simulink model "timeVaryingPathModel3D"  (R2017b)
settings: Solver=VariableStepAuto  StartTime=0.0  StopTime=100  RelTol=1e-3  AbsTol=1e-7
settings Model: Creator=greenoctbass  LastModifiedBy=greenoctbass

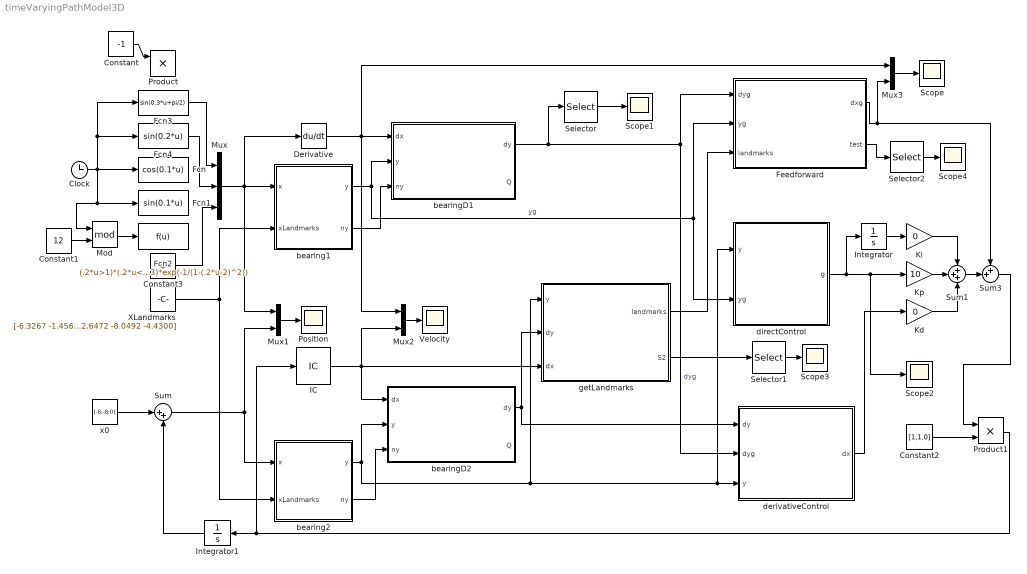
== system timeVaryingPathModel3D ==
  Clock : Clock
  Constant : Constant  Value=-1
  Constant1 : Constant  Value=12
  Constant2 : Constant  Value=[1,1,0]
  Constant3 : Constant  Value=0
  Derivative : Derivative
  Fcn : Fcn  Expr=cos(0.1*u)
  Fcn1 : Fcn  Expr=sin(0.1*u)
  Fcn2 : Fcn  Expr=(.2*u>1)*(.2*u<3)*exp(-1/(1-(.2*u-2)^2))
  Fcn3 : Fcn  Expr=sin(0.3*u+pi/2)
  Fcn4 : Fcn  Expr=sin(0.2*u)
  Feedforward : MATLAB Function  TreatAsAtomicUnit=on
  IC : InitialCondition  Value=[2,2,0]
  Integrator : Integrator
  Integrator1 : Integrator
  Kd : Gain  Gain=0
  Ki : Gain  Gain=0
  Kp : Gain  Gain=10
  Mod : Math  Operator=mod  SaturateOnIntegerOverflow=on
  Mux : Mux  Inputs=3
  Mux1 : Mux  Inputs=2
  Mux2 : Mux  Inputs=2
  Mux3 : Mux  Inputs=2
  Position : Scope
  Product : Product
  Product1 : Product
  Scope{,1..4} (5 alike) : Scope
  Selector : Selector  NumberOfDimensions=2  InputPortWidth=3  IndexOptions=Select all,Index vector (dialog)  Indices=[1 3],2  OutputSizes=1,1
  Selector1 : Selector  InputPortWidth=9  IndexOptions=Index vector (dialog)  Indices=[7 8 9]  OutputSizes=1
  Selector2 : Selector  InputPortWidth=3  IndexOptions=Select all  Indices=[1 2 3]  OutputSizes=1
  Sum : Sum  Inputs=|++
  Sum1 : Sum  Inputs=+++
  Sum3 : Sum  Inputs=++|
  Velocity : Scope
  XLandmarks : Constant  Value=[-6.3267 -1.4564 6.4309 -9.4093 -5.0582 -1.3374; -5.6740 9.4115 -2.6130 -6.1627 1.3438 2.2212; 8.1158 -7.4603 8.2675 2.6472 -8.0492 -4.4300]
  bearing1 : MATLAB Function  TreatAsAtomicUnit=on
  bearing2 : MATLAB Function  TreatAsAtomicUnit=on
  bearingD1 : MATLAB Function  TreatAsAtomicUnit=on
  bearingD2 : MATLAB Function  TreatAsAtomicUnit=on
  derivativeControl : MATLAB Function  TreatAsAtomicUnit=on
  directControl : MATLAB Function  TreatAsAtomicUnit=on
  getLandmarks : MATLAB Function  TreatAsAtomicUnit=on
  x0 : Constant  Value=[-8;-8;0]
  wires:
  XLandmarks/1 -> bearing2/2(xLandmarks), bearing1/2(xLandmarks)
  Mux/1 -> Mux1/1, Derivative/1, bearing1/1(x)
  bearing1/1(y) -> Feedforward/2(yg), directControl/2(yg), bearingD1/2(y)  "yg"
  Derivative/1 -> Mux3/1, bearingD1/1(dx), Mux2/1
  bearing1/2(ny) -> bearingD1/3(ny)
  x0/1 -> Sum/1
  Sum/1 -> Mux1/2, bearing2/1(x)
  bearing2/2(ny) -> bearingD2/3(ny)
  directControl/1(g) -> Integrator/1, Scope2/1, Kp/1
  Integrator/1 -> Ki/1
  Kp/1 -> Sum1/2
  Ki/1 -> Sum1/1
  Integrator1/1 -> Sum/2
  Mux1/1 -> Position/1
  derivativeControl/1(dx) -> Kd/1
  Mux2/1 -> Velocity/1
  bearing2/1(y) -> bearingD2/2(y), getLandmarks/1(y), directControl/1(y), derivativeControl/3(y)
  bearingD1/1(dy) -> derivativeControl/2(dyg), Feedforward/1(dyg), Selector/1  "dyg"
  bearingD2/1(dy) -> getLandmarks/2(dy), derivativeControl/1(dy)
  Kd/1 -> Sum1/3
  Selector/1 -> Scope1/1
  Mux3/1 -> Scope/1
  Product1/1 -> IC/1, Integrator1/1
  Clock/1 -> Mod/1, Fcn1/1, Fcn/1, Fcn4/1, Fcn3/1
  Constant1/1 -> Mod/2
  Constant/1 -> Product/1
  IC/1 -> getLandmarks/3(dx), Mux2/2, bearingD2/1(dx)
  Sum1/1 -> Sum3/2
  Feedforward/1(dxg) -> Sum3/1, Mux3/2
  Mod/1 -> Fcn2/1
  Fcn3/1 -> Mux/1
  Fcn4/1 -> Mux/2
  getLandmarks/1(landmarks) -> Feedforward/3(landmarks)
  getLandmarks/2(S2) -> Selector1/1
  Selector1/1 -> Scope3/1
  Sum3/1 -> Product1/1
  Constant2/1 -> Product1/2
  Constant3/1 -> Mux/3
  Selector2/1 -> Scope4/1
  Feedforward/2(test) -> Selector2/1

== matlab function timeVaryingPathModel3D/bearingD1 ==
  data: dx input; dy output; y input; ny input; Q output
%Compute derivative of bearing vectors
%function [dy,Q]=bearingComputeDerivative(dx,y,ny)
%Inputs
%   dx   derivative of robot's location
%   y   current bearings
%   ny  ranges corresponding to the bearings
%Output
%   dy  derivative of Y along v
%   Q   array of matrices such that dY=Q*v
function [dy,Q]=bearingComputeDerivative(dx,y,ny)
flagComputeQ=false;
if nargout>1
    flagComputeQ=true;
end
[d,Ny]=size(y);
dy=zeros(d,Ny);
if flagComputeQ
    Q=zeros(d,d,Ny);
end
I=eye(d);
for iY=1:Ny
    Qi=-inv(ny(iY))*(I-y(:,iY)*y(:,iY)');
    dy(:,iY)=Qi*dx;
    if flagComputeQ
        Q(:,:,iY)=Qi;
    end
end

== matlab function timeVaryingPathModel3D/bearing1 ==
  data: x input; y output; xLandmarks input; ny output
%Compute bearing information from base point and landmarks
%function [y,ny]=bearingCompute(x,xLandmarks)
%Inputs
%   x           coordinates of base point
%   xLandmarks  coordinates of landmarks
%Outputs
%   y       bearings
%   ny      ranges corresponding to the bearings
%
function [y,ny]=bearingCompute(x,xLandmarks)
Nx=size(x,2);
NxLandmarks=size(xLandmarks,2);
if Nx==1 && NxLandmarks>1
    z=x*ones(1,NxLandmarks);
elseif NxLandmarks==1 && Nx>1
    xLandmarks=xLandmarks*ones(1,Nx);
end
[y,ny]=cnormalize(xLandmarks-z);

== matlab function timeVaryingPathModel3D/bearing2 ==
  data: x input; y output; xLandmarks input; ny output
%Compute bearing information from base point and landmarks
%function [y,ny]=bearingCompute(x,xLandmarks)
%Inputs
%   x           coordinates of base point
%   xLandmarks  coordinates of landmarks
%Outputs
%   y       bearings
%   ny      ranges corresponding to the bearings
%
function [y,ny]=bearingCompute(x,xLandmarks)
Nx=size(x,2);
NxLandmarks=size(xLandmarks,2);
if Nx==1 && NxLandmarks>1
    z=x*ones(1,NxLandmarks);
elseif NxLandmarks==1 && Nx>1
    xLandmarks=xLandmarks*ones(1,Nx);
end
[y,ny]=cnormalize(xLandmarks-z);

== matlab function timeVaryingPathModel3D/bearingD2 ==
  data: dx input; dy output; y input; ny input; Q output
%Compute derivative of bearing vectors
%function [dy,Q]=bearingComputeDerivative(dx,y,ny)
%Inputs
%   dx   derivative of robot's location
%   y   current bearings
%   ny  ranges corresponding to the bearings
%Output
%   dy  derivative of Y along v
%   Q   array of matrices such that dY=Q*v
function [dy,Q]=bearingComputeDerivative(dx,y,ny)
flagComputeQ=false;
if nargout>1
    flagComputeQ=true;
end
[d,Ny]=size(y);
dy=zeros(d,Ny);
if flagComputeQ
    Q=zeros(d,d,Ny);
end
I=eye(d);
for iY=1:Ny
    Qi=-inv(ny(iY))*(I-y(:,iY)*y(:,iY)');
    dy(:,iY)=Qi*dx;
    if flagComputeQ
        Q(:,:,iY)=Qi;
    end
end

== matlab function timeVaryingPathModel3D/directControl ==
  data: y input; g output; yg input
%Compute the velocity control from the bearing potential
%function dx=bearingControlDirect(y,yg,funs)
%Inputs
%   y       Current bearing vectors
%   yg      Goal's bearing vectors
%   funs    Reshaping function for the generalized cost
%
function g=bearingControlDirect(y,yg)
flagPrecondition=false;
funs=bearingCostFunctions('cosine');

%optional parameters
% ivarargin=1;
% while ivarargin<=length(varargin)
%     switch lower(varargin{ivarargin})
%         case 'precondition'
%             flagPrecondition=true;
%         otherwise
%             disp(varargin{ivarargin})
%             error('Argument not valid!')
%     end
%     ivarargin=ivarargin+1;
% end

if ~flagPrecondition
    g=-bearingCostGeneral_gradient_noOptional(y,yg,funs);
else
    g=bearingCostGeneral_gradient(y,yg,funs);
    [~,Hdx]=bearingCostGeneral_gradient_noOptional(y,yg,funs);
    %Hdx=Hdx/det(Hdx);
    g=-Hdx\g;
end

== matlab function timeVaryingPathModel3D/derivativeControl ==
  data: dy input; dx output; dyg input; y input
function dx = bearingControlDerivative(dy,dyg,y)

[d,Ny]=size(y);
I=eye(d);
Q=zeros(d*Ny,d);
Y=zeros(d*Ny,1);
for iY=1:Ny
    Qi=(I-y(:,iY)*y(:,iY)');
    Y((iY-1)*d+1:d*iY)=Qi*(dy(:,iY)-dyg(:,iY));
    Q(((iY-1)*d+1:d*iY),1:d)=Qi;
end
dx=Q\Y;

== matlab function timeVaryingPathModel3D/Feedforward ==
  data: dxg output; dyg input; yg input; landmarks input; test output
%Only works for 2d right now - not really, fix it
function [dxg,test]  = bearingComputeFeedforward(dyg,yg,landmarks)
[d,Ny]=size(landmarks);
I=eye(d);
xg=zeros(d,1);
dxg=xg;
ny=zeros(Ny,1);

if d==3
    A=[yg(2,:)' -yg(1,:)' ny; yg(3,:)' ny -yg(1,:)'];
    temp=[landmarks landmarks];
else
    A=fliplr(yg');
    temp=landmarks;
    A(:,d)=-A(:,d);
end
b=sum(A.*temp',2);
xg=A\b;
points=zeros(size(temp));
for i=1:Ny
    landmarks(:,i)=landmarks(:,i)-xg;
    points(:,i)=dyg(:,i).*norm(landmarks(:,i));
end
if d==3
    points=[points(:,1:Ny) points(:,1:Ny)];
end
b2=sum(A.*-points',2);
dxg=A\b2;

C=zeros(d*Ny,d+Ny);
I=eye(d);
for iY=1:Ny
    Qi=(I-yg(:,iY)*yg(:,iY)');
    C(1+d*(iY-1):d*iY,1:d)=Qi;
    C(1+d*(iY-1):d*iY,iY+d)=dyg(:,iY);
end
[~,S,V]=svd(C,'econ');
NS=V(:,end);
if NS(d+1)<0
    NS=-NS;
end
test=NS(1:d,:);

== matlab function timeVaryingPathModel3D/getLandmarks ==
  data: y input; landmarks output; dy input; dx input; S2 output
%Estimate dx and distances to landmarks for dy and Q matrices.
% function [dx,ny]=bearingComputeSVDEstimate(y,dy)
%Inputs
%   y current bearings
%   dy current derivative of bearings (bearingComputeDerivative)
%Outputs
%   dx current estimated derivative of robot's location
%   ny current estimated distances from landmarks
function [landmarks,S2]  = bearingComputeSVDEstimate(y,dy,dx)
[d,Ny]=size(y);
A=zeros(d*Ny,d+Ny);
I=eye(d);
landmarks=zeros(d,Ny);
for iY=1:Ny
    Qi=(I-y(:,iY)*y(:,iY)');
    A(1+d*(iY-1):d*iY,1:d)=Qi;
    A(1+d*(iY-1):d*iY,iY+d)=dy(:,iY);
end
[~,S,V]=svd(A,'econ');
NS=V(:,Ny+1:end);
alpha=NS(1:d,:)\dx;
v1=NS*alpha;
for i=1:d
    landmarks(i,:)=v1(d+1:end)';
end
landmarks=y.*landmarks;
S2=sum(S,1);
